simulink model "lateral_naolinear"  (R2019b)
settings: Solver=FixedStepAuto  StartTime=0.0  StopTime=2  FixedStep=1e-3  RelTol=1e-3
undefined symbols (not defined in the file): Kpsi, Ky, psi0, psirMax, v, y0, yr
settings Model: Creator=mmaximo  LastModifiedBy=rodri

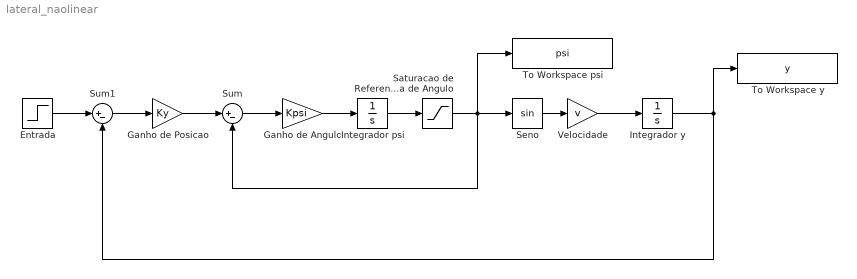
== system lateral_naolinear ==
  Entrada : Step  Time=0  After=yr  SampleTime=0
  Ganho de Angulo : Gain  Gain=Kpsi
  Ganho de Posicao : Gain  Gain=Ky
  Integrador psi : Integrator  InitialCondition=psi0
  Integrador y : Integrator  InitialCondition=y0
  Saturacao de Referencia de Angulo : Saturate  UpperLimit=psirMax  LowerLimit=-psirMax
  Seno : Trigonometry
  Sum : Sum  Inputs=|+-
  Sum1 : Sum  Inputs=|+-
  To Workspace psi : ToWorkspace  VariableName=psi  SaveFormat=Structure With Time  SampleTime=-1
  To Workspace y : ToWorkspace  VariableName=y  SaveFormat=Structure With Time  SampleTime=-1
  Velocidade : Gain  Gain=v
  wires:
  Entrada/1 -> Sum1/1
  Integrador y/1 -> Sum1/2, To Workspace y/1
  Sum1/1 -> Ganho de Posicao/1
  Ganho de Posicao/1 -> Sum/1
  Integrador psi/1 -> Saturacao de Referencia de Angulo/1
  Sum/1 -> Ganho de Angulo/1
  Ganho de Angulo/1 -> Integrador psi/1
  Seno/1 -> Velocidade/1
  Velocidade/1 -> Integrador y/1
  Saturacao de Referencia de Angulo/1 -> Sum/2, To Workspace psi/1, Seno/1
